simulink model "UAM_centralized"  (R2024b)
settings: Solver=VariableStepAuto  StartTime=0.0  StopTime=20  RelTol=1e-3
InitFcn:
  | %% INITIALIZATION
  | UAM_initialization
values from neighbouring files (symbols this model uses):
  csi_dot_init = zeros(9,1)    [UAM_initialization.m]
  csi_init = [p_b_init; eta_b_init; q_init]    [UAM_initialization.m]
  H_b = sym('H_b', [3 3], 'real')    [C_matrix.m]    (also in UAM_initialization.m = diag([1.24, 1.24, 2.48]))
  H_l1 = sym('H_l1', [3 3], 'real')    [C_matrix.m]    (also in C_matrix_manipulator.m; UAM_initialization.m = diag([0, 0, 0]))
  H_l2 = sym('H_l2', [3 3], 'real')    [C_matrix.m]    (also in C_matrix_manipulator.m; UAM_initialization.m = diag([0, 0, 0.0011]))
  H_l3 = sym('H_l3', [3 3], 'real')    [C_matrix.m]    (also in C_matrix_manipulator.m; UAM_initialization.m = diag([0, 0, 1.25e-4]))
  l1 = 0.15    [UAM_initialization.m]
  l2 = 0.05    [UAM_initialization.m]
  m_b = 2.0    (= 2)    [UAM_initialization.m]
  m_l1 = 0    [UAM_initialization.m]
  m_l2 = 0.049    [UAM_initialization.m]
  m_l3 = 0.05    [UAM_initialization.m]
  offset = 0.1    [UAM_initialization.m]
  Ts = 0.001    [UAM_initialization.m]
libraries: simulink x2, cstblocks x2, simulink_extras x1
settings Model: Creator=giuli  LastModifiedBy=giuli

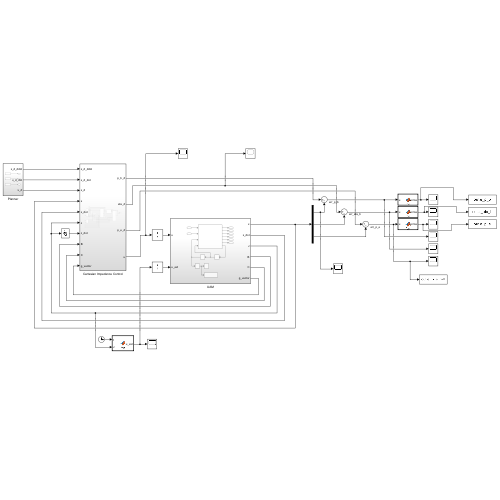
[thumbnail: Simulink's stored preview of the top-level diagram]
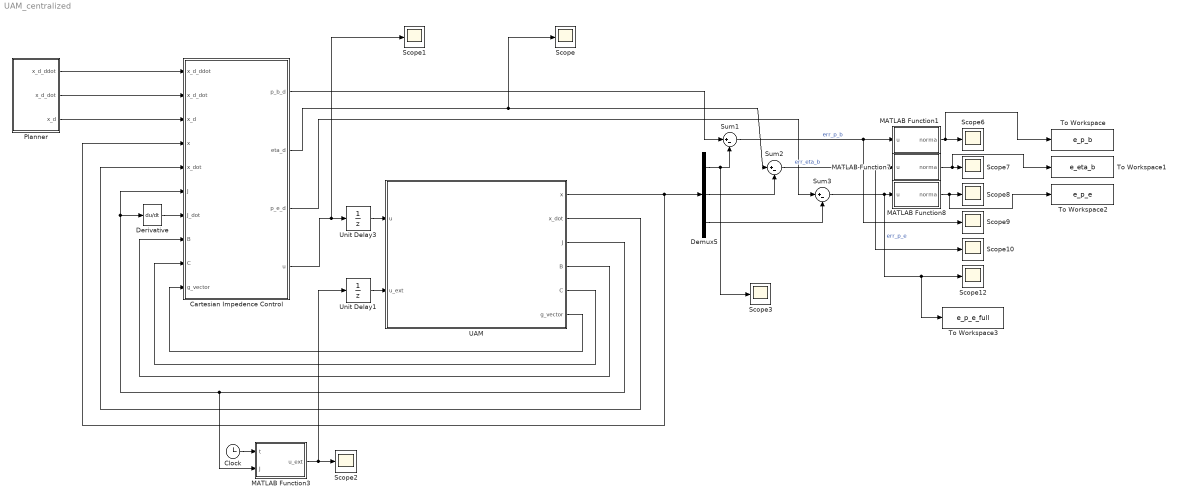
== system UAM_centralized ==
  Cartesian Impedence Control : Subsystem
  Clock : Clock
      settings: Decimation=100
  Demux5 : Demux  Outputs=[3 3 3]
  Derivative : Derivative
  MATLAB Function1 : MATLAB Function  TreatAsAtomicUnit=on
  MATLAB Function3 : MATLAB Function  TreatAsAtomicUnit=on
  MATLAB Function7 : MATLAB Function  TreatAsAtomicUnit=on
  MATLAB Function8 : MATLAB Function  TreatAsAtomicUnit=on
  Planner : Subsystem
  Scope{,1..3,6..10,12} (10 alike) : Scope
  Sum1 : Sum  Inputs=|+-
  Sum2 : Sum  Inputs=|+-
  Sum3 : Sum  Inputs=|+-
  To Workspace : ToWorkspace  VariableName=e_p_b  SampleTime=-1
  To Workspace1 : ToWorkspace  VariableName=e_eta_b  SampleTime=-1
  To Workspace2 : ToWorkspace  VariableName=e_p_e  SampleTime=-1
  To Workspace3 : ToWorkspace  VariableName=e_p_e_full  SampleTime=-1
  UAM : Subsystem
  Unit Delay1 : UnitDelay  SampleTime=Ts  HasFrameUpgradeWarning=on
  Unit Delay3 : UnitDelay  InitialCondition=[(m_b+m_l1+m_l2+m_l3)*9.81;0;0;0;0;0;0]  SampleTime=Ts  HasFrameUpgradeWarning=on
  wires:
  MATLAB Function3/1(u_ext) -> Unit Delay1/1, Scope2/1
  Clock/1 -> MATLAB Function3/1(t)
  UAM/4(B) -> Cartesian Impedence Control/8(B)
  UAM/5(C) -> Cartesian Impedence Control/9(C)
  UAM/6(g_vector) -> Cartesian Impedence Control/10(g_vector)
  UAM/1(x) -> Demux5/1, Cartesian Impedence Control/4(x)
  UAM/3(J) -> MATLAB Function3/2(J), Derivative/1, Cartesian Impedence Control/6(J)
  Unit Delay3/1 -> UAM/1(u)
  Planner/1(x_d_ddot) -> Cartesian Impedence Control/1(x_d_ddot)
  Planner/2(x_d_dot) -> Cartesian Impedence Control/2(x_d_dot)
  Planner/3(x_d) -> Cartesian Impedence Control/3(x_d)
  Derivative/1 -> Cartesian Impedence Control/7(J_dot)
  UAM/2(x_dot) -> Cartesian Impedence Control/5(x_dot)
  Cartesian Impedence Control/2(eta_d) -> Scope/1, Sum2/1
  Cartesian Impedence Control/4(u) -> Scope1/1, Unit Delay3/1
  Cartesian Impedence Control/1(p_b_d) -> Sum1/1
  Cartesian Impedence Control/3(p_e_d) -> Sum3/1
  Demux5/1 -> Scope3/1, Sum1/2
  Demux5/2 -> Sum2/2
  Demux5/3 -> Sum3/2
  Sum1/1 -> Scope9/1, MATLAB Function1/1(u)  "err_p_b"
  Sum2/1 -> Scope10/1, MATLAB Function7/1(u)  "err_eta_b"
  Sum3/1 -> To Workspace3/1, Scope12/1, MATLAB Function8/1(u)  "err_p_e"
  MATLAB Function1/1(norma) -> To Workspace/1, Scope6/1
  MATLAB Function7/1(norma) -> To Workspace1/1, Scope7/1
  MATLAB Function8/1(norma) -> To Workspace2/1, Scope8/1
  Unit Delay1/1 -> UAM/2(u_ext)

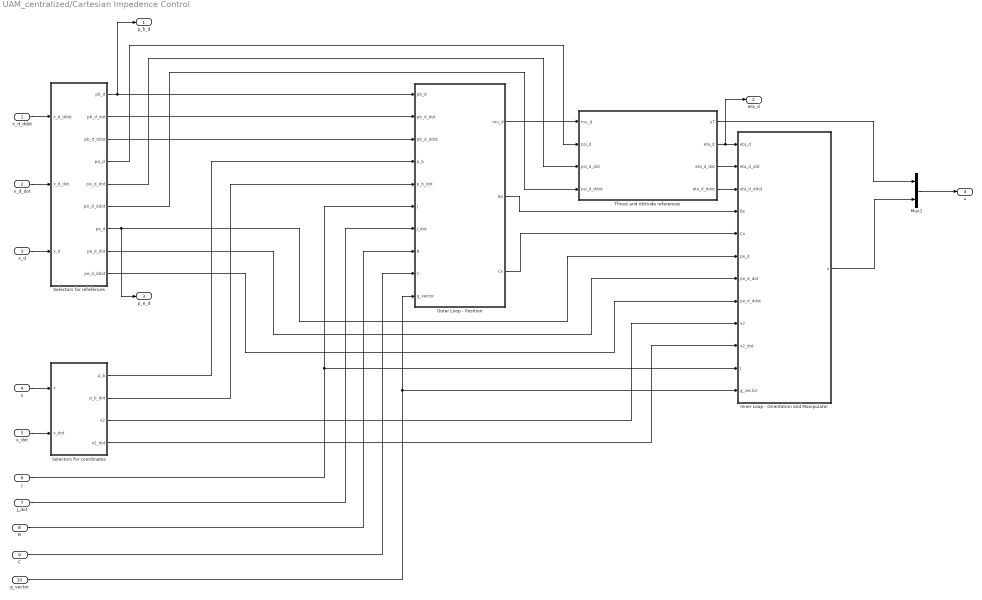
== system UAM_centralized/Cartesian Impedence Control ==
  x_d_ddot : Inport
  x_d_dot : Inport  Port=2
  x_d : Inport  Port=3
  x : Inport  Port=4
  x_dot : Inport  Port=5
  J : Inport  Port=6
  J_dot : Inport  Port=7
  B : Inport  Port=8
  C : Inport  Port=9
  g_vector : Inport  Port=10
  Inner Loop - Orientation and Manipulator : MATLAB Function  TreatAsAtomicUnit=on
  Mux1 : Mux  Inputs=[1 6]
  Outer Loop - Position : MATLAB Function  TreatAsAtomicUnit=on
  Selectors for coordinates : Subsystem
  Selectors for refefences : Subsystem
  Thrust and Attitude references : Subsystem
  p_b_d : Outport
  eta_d : Outport  Port=2
  p_e_d : Outport  Port=3
  u : Outport  Port=4
  wires:
  Outer Loop - Position/2(Bx) -> Inner Loop - Orientation and Manipulator/4(Bx)
  Selectors for refefences/9(pe_d_ddot) -> Inner Loop - Orientation and Manipulator/8(pe_d_ddot)
  Inner Loop - Orientation and Manipulator/1(u) -> Mux1/2
  Selectors for refefences/7(pe_d) -> p_e_d/1, Inner Loop - Orientation and Manipulator/6(pe_d)
  J_dot/1 -> Outer Loop - Position/7(J_dot)
  J/1 -> Inner Loop - Orientation and Manipulator/11(J), Outer Loop - Position/6(J)
  Mux1/1 -> u/1
  Selectors for refefences/4(psi_d) -> Thrust and Attitude references/2(psi_d)
  Thrust and Attitude references/3(eta_d_dot) -> Inner Loop - Orientation and Manipulator/2(eta_d_dot)
  Outer Loop - Position/3(Cx) -> Inner Loop - Orientation and Manipulator/5(Cx)
  Thrust and Attitude references/1(uT) -> Mux1/1
  Outer Loop - Position/1(mu_d) -> Thrust and Attitude references/1(mu_d)
  Selectors for refefences/8(pe_d_dot) -> Inner Loop - Orientation and Manipulator/7(pe_d_dot)
  Selectors for refefences/2(pb_d_dot) -> Outer Loop - Position/2(pb_d_dot)
  Selectors for refefences/6(psi_d_ddot) -> Thrust and Attitude references/4(psi_d_ddot)
  Selectors for refefences/5(psi_d_dot) -> Thrust and Attitude references/3(psi_d_dot)
  Selectors for coordinates/4(x2_dot) -> Inner Loop - Orientation and Manipulator/10(x2_dot)
  g_vector/1 -> Inner Loop - Orientation and Manipulator/12(g_vector), Outer Loop - Position/10(g_vector)
  Thrust and Attitude references/4(eta_d_ddot) -> Inner Loop - Orientation and Manipulator/3(eta_d_ddot)
  Selectors for refefences/1(pb_d) -> p_b_d/1, Outer Loop - Position/1(pb_d)
  Selectors for refefences/3(pb_d_ddot) -> Outer Loop - Position/3(pb_d_ddot)
  Selectors for coordinates/2(p_b_dot) -> Outer Loop - Position/5(p_b_dot)
  x/1 -> Selectors for coordinates/1(x)
  Thrust and Attitude references/2(eta_d) -> eta_d/1, Inner Loop - Orientation and Manipulator/1(eta_d)
  Selectors for coordinates/1(p_b) -> Outer Loop - Position/4(p_b)
  Selectors for coordinates/3(x2) -> Inner Loop - Orientation and Manipulator/9(x2)
  x_d_ddot/1 -> Selectors for refefences/1(x_d_ddot)
  x_d_dot/1 -> Selectors for refefences/2(x_d_dot)
  x_d/1 -> Selectors for refefences/3(x_d)
  x_dot/1 -> Selectors for coordinates/2(x_dot)
  B/1 -> Outer Loop - Position/8(B)
  C/1 -> Outer Loop - Position/9(C)

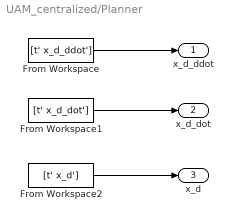
== system UAM_centralized/Planner ==
  From Workspace : FromWorkspace  VariableName=[t' x_d_ddot']  SampleTime=Ts
  From Workspace1 : FromWorkspace  VariableName=[t' x_d_dot']  SampleTime=Ts
  From Workspace2 : FromWorkspace  VariableName=[t' x_d']  SampleTime=Ts
  x_d_ddot : Outport
  x_d_dot : Outport  Port=2
  x_d : Outport  Port=3
  wires:
  From Workspace/1 -> x_d_ddot/1
  From Workspace2/1 -> x_d/1
  From Workspace1/1 -> x_d_dot/1

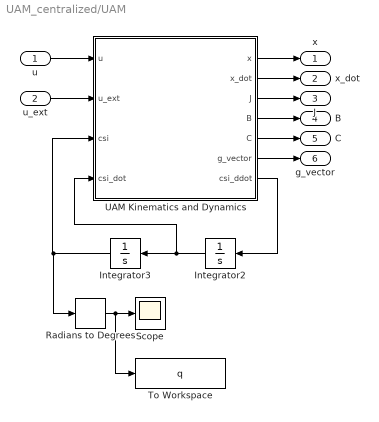
== system UAM_centralized/UAM ==
  u : Inport
  u_ext : Inport  Port=2
  Integrator2 : Integrator  InitialCondition=csi_dot_init
  Integrator3 : Integrator  InitialCondition=csi_init
  Radians to Degrees : simulink_extras/Transformations/Radians to Degrees
  Scope : Scope
  To Workspace : ToWorkspace  VariableName=q  SampleTime=-1
  UAM Kinematics and Dynamics : MATLAB Function  TreatAsAtomicUnit=on
  x : Outport
  x_dot : Outport  Port=2
  J : Outport  Port=3
  B : Outport  Port=4
  C : Outport  Port=5
  g_vector : Outport  Port=6
  wires:
  u_ext/1 -> UAM Kinematics and Dynamics/2(u_ext)
  UAM Kinematics and Dynamics/6(g_vector) -> g_vector/1
  u/1 -> UAM Kinematics and Dynamics/1(u)
  UAM Kinematics and Dynamics/3(J) -> J/1
  UAM Kinematics and Dynamics/4(B) -> B/1
  UAM Kinematics and Dynamics/5(C) -> C/1
  UAM Kinematics and Dynamics/1(x) -> x/1
  UAM Kinematics and Dynamics/2(x_dot) -> x_dot/1
  Integrator2/1 -> UAM Kinematics and Dynamics/4(csi_dot), Integrator3/1
  UAM Kinematics and Dynamics/7(csi_ddot) -> Integrator2/1
  Integrator3/1 -> Radians to Degrees/1, UAM Kinematics and Dynamics/3(csi)
  Radians to Degrees/1 -> To Workspace/1, Scope/1

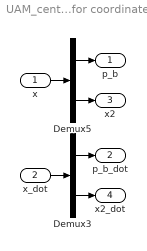
== system UAM_centralized/Cartesian Impedence Control/Selectors for coordinates ==
  x : Inport
  x_dot : Inport  Port=2
  Demux3 : Demux  Outputs=[3 6]
  Demux5 : Demux  Outputs=[3 6]
  p_b : Outport
  p_b_dot : Outport  Port=2
  x2 : Outport  Port=3
  x2_dot : Outport  Port=4
  wires:
  Demux3/2 -> x2_dot/1
  Demux3/1 -> p_b_dot/1
  x_dot/1 -> Demux3/1
  x/1 -> Demux5/1
  Demux5/1 -> p_b/1
  Demux5/2 -> x2/1

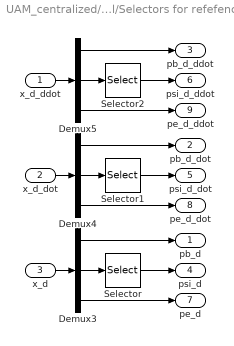
== system UAM_centralized/Cartesian Impedence Control/Selectors for refefences ==
  x_d_ddot : Inport
  x_d_dot : Inport  Port=2
  x_d : Inport  Port=3
  Demux3 : Demux  Outputs=[3 3 3]
  Demux4 : Demux  Outputs=[3 3 3]
  Demux5 : Demux  Outputs=[3 3 3]
  Selector : Selector  InputPortWidth=3  IndexOptions=Index vector (dialog)  Indices=3  OutputSizes=1
  Selector1 : Selector  InputPortWidth=3  IndexOptions=Index vector (dialog)  Indices=3  OutputSizes=1
  Selector2 : Selector  InputPortWidth=3  IndexOptions=Index vector (dialog)  Indices=3  OutputSizes=1
  pb_d : Outport
  pb_d_dot : Outport  Port=2
  pb_d_ddot : Outport  Port=3
  psi_d : Outport  Port=4
  psi_d_dot : Outport  Port=5
  psi_d_ddot : Outport  Port=6
  pe_d : Outport  Port=7
  pe_d_dot : Outport  Port=8
  pe_d_ddot : Outport  Port=9
  wires:
  Demux5/2 -> Selector2/1
  Selector/1 -> psi_d/1
  Demux3/2 -> Selector/1
  Demux4/2 -> Selector1/1
  Selector2/1 -> psi_d_ddot/1
  x_d_dot/1 -> Demux4/1
  x_d_ddot/1 -> Demux5/1
  Demux3/1 -> pb_d/1
  x_d/1 -> Demux3/1
  Demux3/3 -> pe_d/1
  Demux5/3 -> pe_d_ddot/1
  Demux5/1 -> pb_d_ddot/1
  Demux4/1 -> pb_d_dot/1
  Demux4/3 -> pe_d_dot/1
  Selector1/1 -> psi_d_dot/1

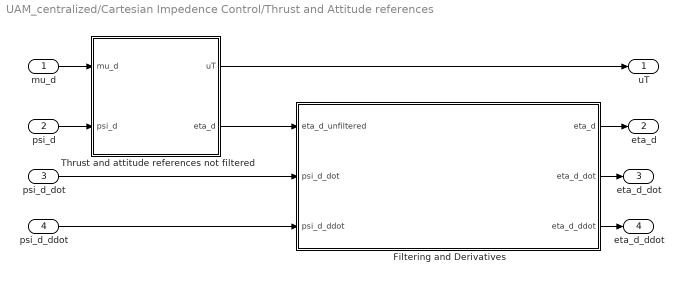
== system UAM_centralized/Cartesian Impedence Control/Thrust and Attitude references ==
  mu_d : Inport
  psi_d : Inport  Port=2
  psi_d_dot : Inport  Port=3
  psi_d_ddot : Inport  Port=4
  Filtering and Derivatives : Subsystem
  Thrust and attitude references not filtered : MATLAB Function  TreatAsAtomicUnit=on
  uT : Outport
  eta_d : Outport  Port=2
  eta_d_dot : Outport  Port=3
  eta_d_ddot : Outport  Port=4
  wires:
  Thrust and attitude references not filtered/1(uT) -> uT/1
  psi_d/1 -> Thrust and attitude references not filtered/2(psi_d)
  Filtering and Derivatives/2(eta_d_dot) -> eta_d_dot/1
  psi_d_ddot/1 -> Filtering and Derivatives/3(psi_d_ddot)
  Filtering and Derivatives/1(eta_d) -> eta_d/1
  mu_d/1 -> Thrust and attitude references not filtered/1(mu_d)
  Filtering and Derivatives/3(eta_d_ddot) -> eta_d_ddot/1
  psi_d_dot/1 -> Filtering and Derivatives/2(psi_d_dot)
  Thrust and attitude references not filtered/2(eta_d) -> Filtering and Derivatives/1(eta_d_unfiltered)

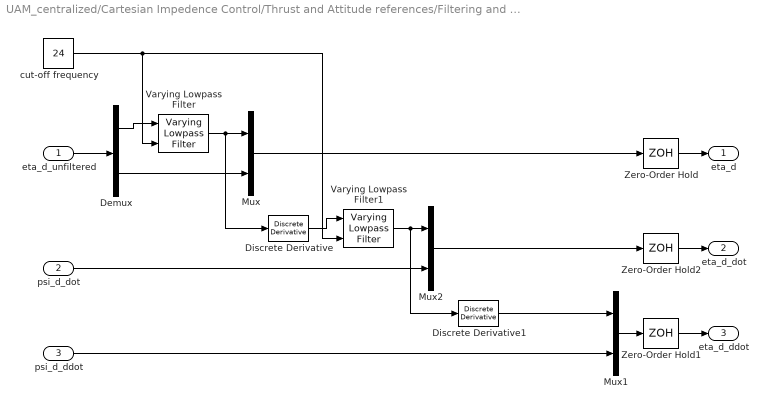
== system UAM_centralized/Cartesian Impedence Control/Thrust and Attitude references/Filtering and Derivatives ==
  eta_d_unfiltered : Inport
  psi_d_dot : Inport  Port=2
  psi_d_ddot : Inport  Port=3
  Demux : Demux  Outputs=[2 1]
  Discrete Derivative : simulink/Discrete/Discrete Derivative  gainval=1.0  ICPrevScaledInput=0.0  OutMin=[]  OutMax=[]  OutDataType=fixdt(1, 16)  OutScaling=2^-10  DoSatur=off
  Discrete Derivative1 : simulink/Discrete/Discrete Derivative  gainval=1.0  ICPrevScaledInput=0.0  OutMin=[]  OutMax=[]  OutDataType=fixdt(1, 16)  OutScaling=2^-10  DoSatur=off
  Mux : Mux  Inputs=[2 1]
  Mux1 : Mux  Inputs=[2 1]
  Mux2 : Mux  Inputs=[2 1]
  Varying Lowpass Filter : cstblocks/Linear Parameter Varying/Varying Lowpass Filter  N=1
  Varying Lowpass Filter1 : cstblocks/Linear Parameter Varying/Varying Lowpass Filter  N=1
  Zero-Order Hold : ZeroOrderHold  SampleTime=Ts
  Zero-Order Hold1 : ZeroOrderHold  SampleTime=Ts
  Zero-Order Hold2 : ZeroOrderHold  SampleTime=Ts
  cut-off frequency : Constant  Value=24
  eta_d : Outport
  eta_d_dot : Outport  Port=2
  eta_d_ddot : Outport  Port=3
  wires:
  Zero-Order Hold2/1 -> eta_d_dot/1
  Zero-Order Hold1/1 -> eta_d_ddot/1
  Zero-Order Hold/1 -> eta_d/1
  Discrete Derivative1/1 -> Mux1/1
  Discrete Derivative/1 -> Varying Lowpass Filter1/1
  psi_d_dot/1 -> Mux2/2
  cut-off frequency/1 -> Varying Lowpass Filter1/2, Varying Lowpass Filter/2
  Varying Lowpass Filter/1 -> Mux/1, Discrete Derivative/1
  Demux/1 -> Varying Lowpass Filter/1
  Demux/2 -> Mux/2
  Varying Lowpass Filter1/1 -> Mux2/1, Discrete Derivative1/1
  psi_d_ddot/1 -> Mux1/2
  eta_d_unfiltered/1 -> Demux/1
  Mux2/1 -> Zero-Order Hold2/1
  Mux1/1 -> Zero-Order Hold1/1
  Mux/1 -> Zero-Order Hold/1

== matlab function UAM_centralized/Cartesian Impedence Control/Thrust and Attitude references/Thrust and attitude references not filtered ==
  data: mu_d input; uT output; psi_d input; eta_d output; m_b parameter; m_l1 parameter; m_l2 parameter; m_l3 parameter
function [uT, eta_d] = fcn(mu_d, psi_d,m_b,m_l1, m_l2, m_l3)
% Compute total thrust and desired attitude from the virtual control input

% Parameters
g = 9.81; 
% m_tot = m_b + m_l1 + m_l2 + m_l3;

% Modified virtual input
mu_bar = mu_d;

% Extract components of mu_bar
mu_bar_1 = mu_bar(1);
mu_bar_2 = mu_bar(2);
mu_bar_3 = mu_bar(3);

% Total Thrust
uT = sqrt(mu_bar_1^2 + mu_bar_2^2 + mu_bar_3^2);

phi_d = asin(1/uT * (-mu_bar_2 * cos(psi_d) + mu_bar_1 * sin(psi_d)));

theta_d = atan((mu_bar_1 * cos(psi_d) + mu_bar_2 * sin(psi_d)) / (mu_bar_3));

% Desired attitude vector
eta_d = [phi_d; theta_d; psi_d];

end

== matlab function UAM_centralized/Cartesian Impedence Control/Inner Loop - Orientation and Manipulator ==
  data: eta_d input; eta_d_dot input; eta_d_ddot input; Bx input; Cx input; pe_d input; pe_d_dot input; pe_d_ddot input; u output; x2 input; x2_dot input; J input; g_vector input
function u = fcn(eta_d,eta_d_dot,eta_d_ddot,  Bx,Cx,  pe_d,pe_d_dot,pe_d_ddot,  x2,x2_dot,  J,g_vector)

% %% Case study A - Rigid Behavior
% Kp = 80 * eye(6);
% zeta = 0.8 * ones(9,1);

%% Case study A - Compliant Behavior
% Kp = 10 * eye(6); %5
% zeta = 0.5 * ones(9,1);

%% Case study B
Kp = blkdiag(20*eye(3),100*eye(3));
zeta = zeros(9,1);                 % Damping ratio
zeta(4:6) = 0.5;
zeta(7:9) = 0.85;

%% Damping
Kp = [zeros(3,6);Kp];
Kd = zeros(9,6);
for i=4:9
    Kd(i,i-3) = 2 * zeta(i) * sqrt(Kp(i,i-3)); 
end

%% Inner Loop Control for orientation and manipulator
% inv_J = inv(J);
% Bx = inv_J' * B * inv_J;
% Cx = inv_J' * (C - B * inv_J * J_dot) * inv_J;

x2_d_ddot = [eta_d_ddot; pe_d_ddot];
x2_d_dot = [eta_d_dot; pe_d_dot];
x2_tilde_dot = [eta_d_dot-x2_dot(1:3); pe_d_dot-x2_dot(4:6)];
x2_tilde = [eta_d-x2(1:3); pe_d-x2(4:6)];

u = g_vector(4:9) + J(1:9, 4:9)' * (Bx(1:9, 4:9) * x2_d_ddot + Cx(1:9, 4:9) * x2_d_dot + Kd * x2_tilde_dot + Kp * x2_tilde);

== matlab function UAM_centralized/MATLAB Function1 ==
  data: u input; norma output
function norma = fcn(u)
norma = norm([u(1);u(2);u(3)]);

== matlab function UAM_centralized/MATLAB Function7 ==
  data: u input; norma output
function norma = fcn(u)
norma = norm([u(1);u(2);u(3)]);

== matlab function UAM_centralized/MATLAB Function8 ==
  data: u input; norma output
function norma = fcn(u)
norma = norm([u(1);u(2);u(3)]);

== matlab function UAM_centralized/MATLAB Function3 ==
  data: t input; J input; u_ext output
function u_ext = fcn(t,J)
A = 1;
omega = pi/2;

if t <= 10
    wind = A*sin(omega*t);

    if wind >= 0
        f_ext = [wind; zeros(8,1)];
    else
        f_ext = zeros(9,1);
    end
else
    f_ext = zeros(9,1);
end

f_ext = [f_ext(1:6); [-0.5; 0; 0]]; % [-0.5; 0; 0]


u_ext = J' * f_ext;

== matlab function UAM_centralized/UAM/UAM Kinematics and Dynamics ==
  data: x output; x_dot output; J output; B output; C output; g_vector output; u input; u_ext input; csi input; csi_ddot output; csi_dot input; m_b parameter; H_b parameter; m_l1 parameter; m_l2 parameter; m_l3 parameter; l1 parameter; l2 parameter; H_l1 parameter; H_l2 parameter; H_l3 parameter; offset parameter
function [x,x_dot,  J,B,C,g_vector,  csi_ddot] = fcn(u, u_ext, csi,csi_dot, m_b, H_b, m_l1, m_l2, m_l3, l1, l2, H_l1, H_l2, H_l3, offset)

% Parameters
g = 9.81;       % gravity acceleration value
e3 = [0;0;1];   % selecting vector

%% State Variables from Generalized Joints Vector (csi)
% Extracting components of the generalized state vector 'csi'
p_b = csi(1:3);    % Position of UAV body frame origin in inertial frame
eta_b = csi(4:6);  % Euler angles (Yaw, Pitch, Roll) of UAV body frame
q = csi(7:9);      % Manipulator joint angles

% Euler angles
phi = eta_b(1);    % Roll angle
theta = eta_b(2);  % Pitch angle
psi = eta_b(3);    % Yaw angle

%% UAV Kinematics: Rotation Matrices and Angular Velocity Mapping
% Individual Rotation Matrices
% Rotation about X-axis (Roll)
Rx = [1,           0,          0;
      0, cos(phi), -sin(phi);
      0, sin(phi),  cos(phi)];

% Rotation about Y-axis (Pitch)
Ry = [cos(theta),  0, sin(theta);
      0,           1,          0;
     -sin(theta),  0, cos(theta)];

% Rotation about Z-axis (Yaw)
Rz = [cos(psi), -sin(psi), 0;
      sin(psi),  cos(psi), 0;
      0,         0,         1];

% Combined Rotation Matrix R_b (from UAV body frame to Inertial frame)
% Using Z-Y-X Euler angle convention (Yaw-Pitch-Roll)
R_b = Rz * Ry * Rx;

% mapping between time derivative of eta_b into UAV angular velocity omega_b_b expressed wrt Sigma_b
Q = [   1     0           -sin(theta);
        0     cos(phi)    cos(theta)*sin(phi);
        0     -sin(phi)   cos(theta)*cos(phi)];    % It's easier to compute first Q

% T_b matrix: Maps Euler angle rates (phi_dot) to body angular velocity (omega_b)
% omega_b = T_b * phi_dot
T_b = R_b * Q;        % it's easier this way

% Q = R_b' * T_b;     

% Ab: Homogeneous transformation matrix from Inertial frame to UAV Body frame
A_b = [R_b,   p_b;
      0 0 0, 1];


%% Manipulator Direct Kinematics (Relative to UAV Body Frame)
% Static Transformation to take into account the offset between UAV and Manipulator
R_b_0 = [1,           0,          0;
        0, cos(pi/2), -sin(pi/2);
        0, sin(pi/2),  cos(pi/2)];  % rotation of pi/2 about x-axis
T_b_0 = [   R_b_0, [0;0;-offset];      % translation along zb
            0,   0,   0,   1];

% D-H parameters for the manipulator
a = [0, l1, l2];
d = [0, 0, 0];
alpha = [pi/2, -pi/2, 0];

% Standard DH transformation matrix A(alpha, a, d, theta) - here theta is q_i
DH_matrix = @(alpha_i, a_i, d_i, q_i) ...
    [cos(q_i), -sin(q_i)*cos(alpha_i),  sin(q_i)*sin(alpha_i),  a_i*cos(q_i);
     sin(q_i),  cos(q_i)*cos(alpha_i), -cos(q_i)*sin(alpha_i),  a_i*sin(q_i);
     0,         sin(alpha_i),          cos(alpha_i),           d_i;
     0,         0,                     0,                      1];

A_0_1 = DH_matrix(alpha(1), a(1), d(1), q(1));
A_1_2 = DH_matrix(alpha(2), a(2), d(2), q(2));
A_2_3 = DH_matrix(alpha(3), a(3), d(3), q(3));

% Transformations from manipulator base frame (Frame 0) to each link frame
T_0_0 = eye(4); % Transformation from Frame 0 to Frame 0
T_0_1 = A_0_1;  % Transformation from Frame 0 to Frame 1
T_0_2 = A_0_1 * A_1_2; % Transformation from Frame 0 to Frame 2
T_0_3 = A_0_1 * A_1_2 * A_2_3; % Transformation from Frame 0 to Frame 3

R_0_0 = T_0_0(1:3, 1:3); p_0_0 = T_0_0(1:3, 4);
R_0_1 = T_0_1(1:3, 1:3); p_0_1 = T_0_1(1:3, 4);
R_0_2 = T_0_2(1:3, 1:3); p_0_2 = T_0_2(1:3, 4);

% Rotation about the y-axis
R_3_e = [cos(pi/2),  0, sin(pi/2);
        0,           1,          0;
        -sin(pi/2),  0, cos(pi/2)];
% To align the z-axis to the approach axis
T_3_e = [R_3_e,         zeros(3,1);
         zeros(1,3),    1];

T_0_e = T_0_3 * T_3_e;

p_0_e = T_0_e(1:3, 4);

% Direct kinematic of the Manipulator from UAV body frame to end-effector frame
A_b_e = T_b_0 * T_0_3 * T_3_e;

% Extract position of end-effector frame origin in UAV body frame (p_b_e)
% p_e^b is position vector of the origin of end-effector frame wrt Sigma_b 
p_b_e = A_b_e(1:3, 4);

%% Absolute Pose of the End-Effector
% A_e: Absolute homogeneous transformation matrix of the end-effector (in Inertial frame)
A_e = A_b * A_b_e;

%R_e = A_e(1:3, 1:3);

% Extract p_e (position of end-effector in inertial frame)
p_e = A_e(1:3, 4); % This is p_e from x = [p_b^T, eta_b^T, p_e^T]^T 

x = [p_b; eta_b; p_e];

%% Manipulator Jacobian (in manipulator 0 frame)
% For revolute joints
% JPi = z_{i-1} X (p_e - p_{i-1})
% JOi = z_{i-1}

% z_{i-1} is the third column of the rotation matrix R_0_{i-1}
z_0 = R_0_0(:, 3);
z_1 = R_0_1(:, 3);
z_2 = R_0_2(:, 3);

% Manipulator Translational Jacobian (J_P_0_e) for End-Effector in Frame 0
J_P_0_e = zeros(3,3);
J_P_0_e(:,1) = skew(z_0) * (p_0_e - p_0_0);
J_P_0_e(:,2) = skew(z_1) * (p_0_e - p_0_1);
J_P_0_e(:,3) = skew(z_2) * (p_0_e - p_0_2);

% Manipulator Rotational Jacobian (J_O_0_e) for End-Effector in Frame 0
% J_O_0_e = zeros(3,3);
% J_O_0_e(:,1) = z_0;
% J_O_0_e(:,2) = z_1;
% J_O_0_e(:,3) = z_2;

%% General System Jacobian (J, 9x9 matrix mapping csi_dot to x_dot)
% csi_dot = [p_b_dot; eta_b_dot; q_dot]
% x_dot = [p_b_dot; eta_b_dot; p_e_dot]
J = zeros(9,9);

% --- Row Block 1 (for p_b_dot = p_b_dot) ---
J(1:3, 1:3) = eye(3);
J(1:3, 4:6) = zeros(3); % No dependence on eta_b_dot
J(1:3, 7:9) = zeros(3); % No dependence on q_dot

% --- Row Block 2 (for eta_b_dot = eta_b_dot) ---
J(4:6, 1:3) = zeros(3); % No dependence on p_b_dot
J(4:6, 4:6) = eye(3);
J(4:6, 7:9) = zeros(3); % No dependence on q_dot

% --- Row Block 3 (for p_e_dot) ---
% p_e = p_b + R_b * p_b_e
% p_e_dot = p_b_dot + R_b_dot * p_b_e + R_b * p_b_e_dot

% R_b_dot = skew(omega_b) * R_b
% skew(omega_b) * R_b * p_b_e = -skew(R_b * p_b_e) * omega_b     Anti-commutative property
% Using omega_b = T_b * eta_b_dot:
% p_e_dot = p_b_dot - skew(R_b * p_b_e) * T_b * eta_b_dot + R_b * R_b_0 * J_P_0_e * q_dot
J(7:9, 1:3) = eye(3);                        % Coefficient of pb_dot
J(7:9, 4:6) = -skew(R_b * p_b_e) * T_b;      % Coefficient of eta_b_dot
J(7:9, 7:9) = R_b * R_b_0 * J_P_0_e;         % Coefficient of q_dot

x_dot = J * csi_dot;

%% Link CoM Transformations and Rotations
% Computation of "p_b_li" which is the position of the center of mass of the link i with respect to UAV body frame (Sigma_b)
% Define Center of Mass (CoM) Positions in the DH's Own Frame
% Remember that the first two joints are in the same point before Link 1
% So let's call the actual Link 1 with "Link 2"
p_0_l1 = [0; 0; 0];
p_1_l2 = [l1/2; 0; 0];
p_2_l3 = [l2/2; 0; 0];

% For Link 1    (It doesn't actually exist)
p_b_0 = T_b_0(1:3, 4);
p_b_l1 = p_b_0 + R_b_0 * p_0_l1;     % Position of the CoM of Link 1 wrt Sigma_b
R_b_l1 = R_b_0;                      % Rotation matrix between the frame associated to the center of mass of the i-th link and Σb

% For Link 2
T_b_1 = T_b_0 * T_0_1;
R_b_1 = T_b_1(1:3, 1:3);
p_b_1 = T_b_1(1:3, 4);
p_b_l2 = p_b_1 + R_b_1 * p_1_l2;     % Position of the CoM of Link 2 wrt Sigma_b
R_b_l2 = R_b_1;

% For Link 2
T_b_2 = T_b_0 * T_0_2;
R_b_2 = T_b_2(1:3, 1:3);
p_b_2 = T_b_2(1:3, 4);
p_b_l3 = p_b_2 + R_b_2 * p_2_l3;     % Position of the CoM of Link 3 wrt Sigma_b
R_b_l3 = R_b_2;

%% Jacobians for Each Link's CoM (wrt Sigma_b)
% For revolute joints
% J_Pj_li = z_{j-1} X (p_com_i - p_{j-1})   % Jacobian for contribution of the first j joints to the linear motion of CoM of Link i
% J_Oj_li = z_{j-1}                         % Jacobian for contribution of the first j joints to the angular motion of CoM of Link i


% z_{j-1} is the third column of the rotation matrix R_b_{j-1}
z_0 = R_b_0(:, 3);
z_1 = R_b_1(:, 3);
z_2 = R_b_2(:, 3);

% Link 1
J_P_l1 = zeros(3,3);
J_P_l1(:,1) = skew(z_0) * (p_b_l1 - p_b_0);

J_O_l1 = zeros(3,3);
J_O_l1(:,1) = z_0;

% Link 2
J_P_l2 = zeros(3,3);
J_P_l2(:,1) = skew(z_0) * (p_b_l2 - p_b_0);
J_P_l2(:,2) = skew(z_1) * (p_b_l2 - p_b_1);

J_O_l2 = zeros(3,3);
J_O_l2(:,1) = z_0;
J_O_l2(:,2) = z_1;

% Link 3
J_P_l3 = zeros(3,3);
J_P_l3(:,1) = skew(z_0) * (p_b_l3 - p_b_0);
J_P_l3(:,2) = skew(z_1) * (p_b_l3 - p_b_1);
J_P_l3(:,3) = skew(z_2) * (p_b_l3 - p_b_2);

J_O_l3 = zeros(3,3);
J_O_l3(:,1) = z_0;
J_O_l3(:,2) = z_1;
J_O_l3(:,3) = z_2;

%% Inertia Matrix B
% B11
B11 = (m_b + m_l1 + m_l2 + m_l3) * eye(3);

% B22
B22_sum_term = m_l1 * T_b' * skew(R_b * p_b_l1)' * skew(R_b * p_b_l1) * T_b + ...
               m_l2 * T_b' * skew(R_b * p_b_l2)' * skew(R_b * p_b_l2) * T_b + ...
               m_l3 * T_b' * skew(R_b * p_b_l3)' * skew(R_b * p_b_l3) * T_b + ...
               Q' * R_b_l1 * H_l1 * R_b_l1' * Q + ... 
               Q' * R_b_l2 * H_l2 * R_b_l2' * Q + ...
               Q' * R_b_l3 * H_l3 * R_b_l3' * Q;
B22 = Q' * H_b * Q + B22_sum_term;

% B33
B33 = (m_l1 * (J_P_l1)' * J_P_l1 + J_O_l1' * R_b_l1 * H_l1 * R_b_l1' * J_O_l1) + ...
      (m_l2 * (J_P_l2)' * J_P_l2 + J_O_l2' * R_b_l2 * H_l2 * R_b_l2' * J_O_l2) + ...
      (m_l3 * (J_P_l3)' * J_P_l3 + J_O_l3' * R_b_l3 * H_l3 * R_b_l3' * J_O_l3);

% B12
B12 = - (m_l1 * skew(R_b * p_b_l1) * T_b + ...
         m_l2 * skew(R_b * p_b_l2) * T_b + ...
         m_l3 * skew(R_b * p_b_l3) * T_b);
B21 = B12';

% B13
B13 = (m_l1 * R_b * J_P_l1) + (m_l2 * R_b * J_P_l2) + (m_l3 * R_b * J_P_l3);
B31 = B13';

% B23
B23_sum1 = Q' * R_b_l1 * H_l1 * R_b_l1' * J_O_l1 + ...
           Q' * R_b_l2 * H_l2 * R_b_l2' * J_O_l2 + ...
           Q' * R_b_l3 * H_l3 * R_b_l3' * J_O_l3;
B23_sum2 = - (m_l1 * T_b' * skew(R_b * p_b_l1)' * R_b * J_P_l1 + ...
              m_l2 * T_b' * skew(R_b * p_b_l2)' * R_b * J_P_l2 + ...
              m_l3 * T_b' * skew(R_b * p_b_l3)' * R_b * J_P_l3);
B23 = B23_sum1 + B23_sum2;
B32 = B23';

% Full B
B = [B11, B12, B13;
     B21, B22, B23;
     B31, B32, B33];

%% Gravity vector contribution g(csi)
% Partial derivative of potential energy U wrt csi
% U = m_b * g * e3' * p_b + sum(m_li * g * e3' * (p_b + R_b * p_b_li))

% Derivative of U wrt p_b
g_pb = ((m_b + m_l1 + m_l2 + m_l3) * g * e3')'; 

% Derivative of U wrt eta_b     (computed using symbolic toolbox)
g_phib = zeros(3,1);
g_phib(1) = g*cos(phi)*cos(theta)*(m_l3*(l1 + l2/2)*(cos(pi/2)^2*sin(q(2)) - sin(q(2)) + cos(pi/2)*cos(q(2))*sin(q(1)) + cos(pi/2)^2*cos(q(1))*sin(q(2))) + (l1*m_l2*cos(pi/2)*sin(q(1)))/2) - g*cos(theta)*sin(phi)*((l1*m_l2*sin(pi/2)*sin(q(1)))/2 - m_l2*offset - m_l3*offset - m_l1*offset + l1*m_l3*sin(pi/2)*cos(q(2))*sin(q(1)) + (l2*m_l3*sin(pi/2)*cos(q(2))*sin(q(1)))/2 + l1*m_l3*cos(pi/2)*sin(pi/2)*sin(q(2)) + (l2*m_l3*cos(pi/2)*sin(pi/2)*sin(q(2)))/2 + l1*m_l3*cos(pi/2)*sin(pi/2)*cos(q(1))*sin(q(2)) + (l2*m_l3*cos(pi/2)*sin(pi/2)*cos(q(1))*sin(q(2)))/2);
g_phib(2) = - g*cos(theta)*((l1*m_l2*cos(q(1)))/2 + l1*m_l3*cos(q(1))*cos(q(2)) + (l2*m_l3*cos(q(1))*cos(q(2)))/2 - l1*m_l3*cos(pi/2)*sin(q(1))*sin(q(2)) - (l2*m_l3*cos(pi/2)*sin(q(1))*sin(q(2)))/2) - g*sin(phi)*sin(theta)*(m_l3*(l1 + l2/2)*(cos(pi/2)^2*sin(q(2)) - sin(q(2)) + cos(pi/2)*cos(q(2))*sin(q(1)) + cos(pi/2)^2*cos(q(1))*sin(q(2))) + (l1*m_l2*cos(pi/2)*sin(q(1)))/2) - g*cos(phi)*sin(theta)*((l1*m_l2*sin(pi/2)*sin(q(1)))/2 - m_l2*offset - m_l3*offset - m_l1*offset + l1*m_l3*sin(pi/2)*cos(q(2))*sin(q(1)) + (l2*m_l3*sin(pi/2)*cos(q(2))*sin(q(1)))/2 + l1*m_l3*cos(pi/2)*sin(pi/2)*sin(q(2)) + (l2*m_l3*cos(pi/2)*sin(pi/2)*sin(q(2)))/2 + l1*m_l3*cos(pi/2)*sin(pi/2)*cos(q(1))*sin(q(2)) + (l2*m_l3*cos(pi/2)*sin(pi/2)*cos(q(1))*sin(q(2)))/2);
g_phib(3) = 0;


% Derivative of U wrt q
% U_manip = sum(m_li * g * e3' * R_b * p_b_li)
% derivative(p_b_li) = J_P_li
sum_m = (m_l1 * J_P_l1 + m_l2 * J_P_l2 + m_l3 * J_P_l3);
g_q = (g * e3' * R_b * sum_m)';

% Full g vector
g_vector = [g_pb; g_phib; g_q];

%% Coriolis matrix C(csi, csi_dot) (using Christoffel symbols of the first type)
% Computed using external script
C = calculate_C_matrix(csi, csi_dot, m_b, m_l1, m_l2, m_l3, l1, l2, offset, H_b, H_l1, H_l2, H_l3, pi);

%% Generelized vector acceleration
% B * csi_ddot + C * csi_dot + g = u + u_ext

% the input u is [uT; tau_b; tau_q]
u2 = [u(1)*R_b*e3; u(2:end)];

csi_ddot = B \ (u2 + u_ext - C * csi_dot - g_vector);

end

function S = skew(v)
    if(numel(v)~= 1)
        S= [0 -v(3) v(2); 
            v(3) 0 -v(1);
            -v(2) v(1) 0];
    else
        S= zeros(3);
    end
end

== matlab function UAM_centralized/Cartesian Impedence Control/Outer Loop - Position ==
  data: mu_d output; Bx output; Cx output; pb_d input; pb_d_dot input; pb_d_ddot input; p_b input; p_b_dot input; J input; J_dot input; B input; C input; g_vector input
function [mu_d, Bx, Cx] = fcn(pb_d, pb_d_dot, pb_d_ddot, p_b, p_b_dot, J,J_dot, B,C,g_vector)

%% Case study A - Rigid Behavior
% Kp = 80 * eye(3);
% zeta = 0.8 * ones(3,1);

%% Case study A - Compliant Behavior
% Kp = 10 * eye(3); %5
% zeta = 0.5 * ones(3,1);

%% Case study B
Kp = 20 * eye(3);
zeta = 0.5 * ones(3,1);

%% Gain matrices
Kp = [Kp; zeros(6,3)];
Kd = zeros(9,3);
for i=1:3
    Kd(i,i) = 2 * zeta(i) * sqrt(Kp(i,i)); 
end

%% Outer Loop Control just for the position
pb_tilde = pb_d - p_b;
pb_tilde_dot = pb_d_dot - p_b_dot;

inv_J = inv(J);
Bx = inv_J' * B * inv_J;
Cx = inv_J' * (C - B * inv_J * J_dot) * inv_J;

mu_d = g_vector(1:3) + J(1:9, 1:3)' * (Bx(1:9, 1:3) * pb_d_ddot + Cx(1:9, 1:3) * pb_d_dot + Kd * pb_tilde_dot + Kp * pb_tilde);
